simulink model "attitude_template_link"  (R2019a)
settings: Solver=ode1  StartTime=0.0  StopTime=inf  FixedStep=1/1000  RelTol=1e-3
PreLoadFcn:
  | x_setpoint_NED = 0;
  | y_setpoint_NED = 0;
  | z_setpoint_NED = 0;
  | vx_setpoint_NED = 0;
  | vy_setpoint_NED = 0;
  | vz_setpoint_NED = 0;
  | afx_setpoint_NED = 0;
  | afy_setpoint_NED = 0;
  | afz_setpoint_NED = 0;
  | yaw_setpoint_NED = 0;
  | yawrate_setpoint_NED = 0;
  | selected_mission = 1;
  | pitch_ol = 0;
  | roll_ol = 0;
  | yaw_ol = 0;
  | theta_xz_setpoint = 0;
  | thrustVal = 0;
  | parentThruster = 0;
  | 
  | return_com = 0;
  | takeoff_com = 0;
  | mission_com = 0;
  | hold_com = 0;
  | land_com = 0;
  | direct_com = 0;
  | origin_update = 0;
InitFcn:
  | x_setpoint_NED = 0;
  | y_setpoint_NED = 0;
  | z_setpoint_NED = 0;
  | vx_setpoint_NED = 0;
  | vy_setpoint_NED = 0;
  | vz_setpoint_NED = 0;
  | afx_setpoint_NED = 0;
  | afy_setpoint_NED = 0;
  | afz_setpoint_NED = 0;
  | yaw_setpoint_NED = 0;
  | yawrate_setpoint_NED = 0;
  | selected_mission = 1;
  | pitch_ol = 0;
  | roll_ol = 0;
  | yaw_ol = 0;
  | theta_xz_setpoint = 0;
  | thrustVal = 0;
  | parentThruster = 0;
  | 
  | return_com = 0;
  | takeoff_com = 0;
  | mission_com = 0;
  | hold_com = 0;
  | land_com = 0;
  | direct_com = 0;
  | origin_update = 0;
StartFcn:
  | yaw_ol = 0;
undefined symbols (not defined in the file or in its folder): f, Object1, Object2, origin_pos_yaw, pitch, roll, roll_input, Standard_Devices, time_usec, UDP_Protocol, x, y, yaw, z
libraries: simulink_extras x17, simulink x3, sldrtlib x3, instrumentlib x1
settings Model: Creator=Admin  LastModifiedBy=viconadmin
settings DataIOCC: SaveFormat=StructureWithTime  ReturnWorkspaceOutputs=off
settings DebuggingCC: ArithmeticOperatorsInVariantConditions=warning
settings SFSimCC: SimUseLocalCustomCode=off
settings RTWCC: RTWUseLocalCustomCode=off
settings CodeAppCC: StateflowObjectComments=on

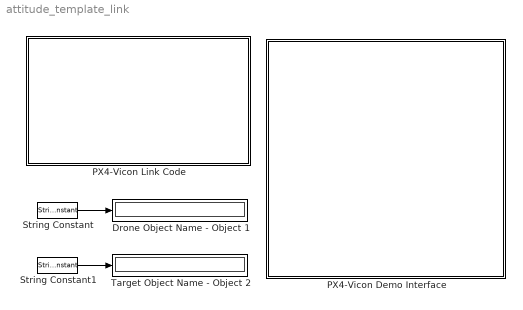
== system attitude_template_link ==
  Drone Object Name - Object 1 : Display
  PX4-Vicon Demo Interface : Subsystem
  PX4-Vicon Link Code : Subsystem
  String Constant : StringConstant  String=Object1
  String Constant1 : StringConstant  String=Object2
  Target Object Name - Object 2 : Display
  wires:
  String Constant/1 -> Drone Object Name - Object 1/1
  String Constant1/1 -> Target Object Name - Object 2/1

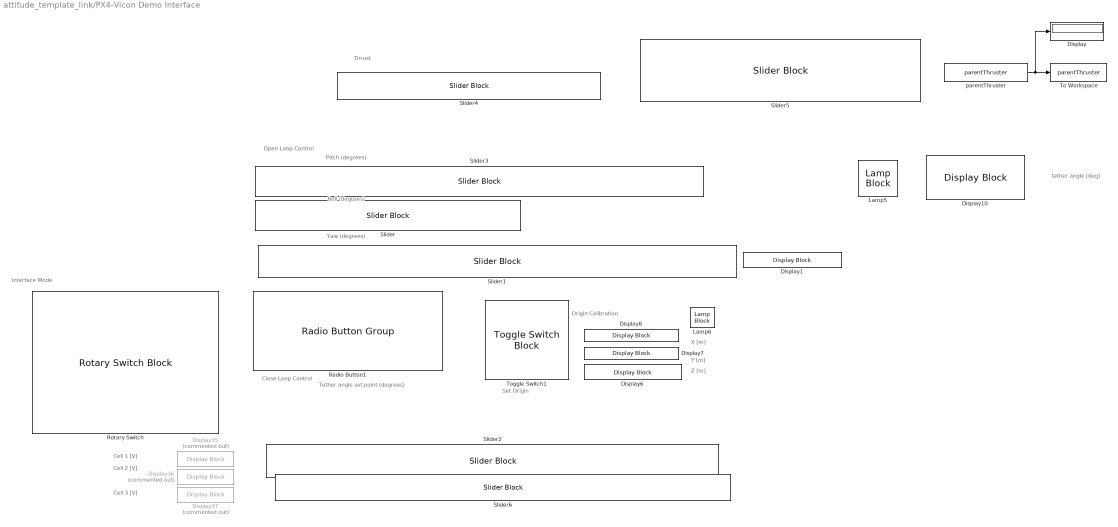
== system attitude_template_link/PX4-Vicon Demo Interface ==
  note: Thrust
  note: Roll (degrees)
  note: Yaw (degrees)
  note: Pitch (degrees)
  note: Interface Mode
  note: Close Loop Control
  note: Cell 1 [V]
  note: Cell 3 [V]
  note: Cell 2 [V]
  note: Set Origin
  note: X [m]
  note: Y [m]
  note: Z [m]
  note: Origin Calibration
  note: Open Loop Control
  note: Tether angle set point (degrees)
  note: tether angle [deg]
  Display : Display
  Display{1,6..8,10} (5 alike) : DisplayBlock  LabelPosition=Hide  Format=short
  Display35 : DisplayBlock  Commented=on  LabelPosition=Hide  Format=short
  Display36 : DisplayBlock  Commented=on  LabelPosition=Hide  Format=short
  Display37 : DisplayBlock  Commented=on  LabelPosition=Hide  Format=short
  Lamp5 : LampBlock
  Lamp6 : LampBlock  LabelPosition=Hide
  Radio Button1 : RadioButtonGroup  LabelPosition=Hide  SelectedLabel=DONT  ButtonGroupName=Select Desired Control
      settings: Values={{'DONT', 'CL control', 'OL Control'}, [1 2 3]}
  Rotary Switch : RotarySwitchBlock  LabelPosition=Hide
      settings: Values={{'Hold Origin', 'Follow', 'Other'}, [1 2 3]}
  Slider : SliderBlock  LabelPosition=Hide  ScaleMin=-25  ScaleMax=25
  Slider1 : SliderBlock  LabelPosition=Hide  ScaleMin=-180  ScaleMax=180  TickInterval=10
  Slider2 : SliderBlock  LabelPosition=Hide  ScaleMin=-30  ScaleMax=60
  Slider3 : SliderBlock  LabelPosition=Hide  ScaleMin=-25  ScaleMax=60  TickInterval=5
  Slider4 : SliderBlock  LabelPosition=Hide  ScaleMax=0.5  TickInterval=0.050000000000000003
  Slider5 : SliderBlock  ScaleMax=60  TickInterval=5
  Slider6 : SliderBlock  LabelPosition=Hide  ScaleMin=-30  ScaleMax=30
  To Workspace : ToWorkspace  VariableName=parentThruster  SaveFormat=Timeseries  SampleTime=-1
  Toggle Switch1 : ToggleSwitchBlock  LabelPosition=Hide
      settings: Values={{'No action', 'Set Origin'}, [0 1]}
  parentThruster : Constant  Value=parentThruster
  wires:
  parentThruster/1 -> Display/1, To Workspace/1

== system attitude_template_link/PX4-Vicon Link Code ==
  note: MAVLink PX4 Interface Telemetry
  note: MAVLink PX4 Interface Motion Capture
  Data Manipulation : Subsystem
  Decode PX4  Telemetry Data - MAVLink : S-Function  FunctionName=sfun_decode_mavlink  SFunctionDeploymentMode=off  EnableBusSupport=off
  Mavlink Encoded - UDP Packet Output : sldrtlib/Packet Output  SampleTime=1/50  MaxMissedTicks=inf  ShowMissedTicks=off  YieldWhenWaiting=off  DrvName=Standard_Devices/UDP_Protocol  DrvAddress=14551  DrvOptions=[0 14556 48 46 48 46 48 46 48 0 0 0 0 0 0 0 0 0 0 0 0 0 0 0 0 0 0 0 0 0 0 0 0 0 0 0 0 0 0 0 0 0 0 0 0 0 0 0 0 0 0 0 0 0 0 0 0 0 0 0 0 0 0 0 0 0 0 0 0 0 0 0 0 0 0 0 0 0 0 0 0 0 0 0 0 0 0 0 0 0 0 0 0 0 0 0 0 0 0 0 0 0 0 0 0 0 0 0 0 0 0 0 0 0 0 0 0 0 0 0 0 0 0 0 0 0 0 0 0 0 0 0 0 0 0 0 0 0 0 0 0 0 0 0 0 0 0 0 0 0 0 0 0 0 0 0 0 0 0 0 0 0 0 0 0 0 0 0 0 0 0 0 0 0 0 0 0 0 0 0 0 0 0 0 0 0 0 0 0 0 0 0 0 0 0 0 0 0 0 0 0 0 0 0 0 0 0 0 0 0 0 0 0 0 0 0 0 0 0 0 0 0 0 0 0 0 0 0 0 0 0 0 0 0 0 0 0 0 0 0 0 0 0 0 0 0 0 0 0 0 0 0 0 0 0 0]  PacketSize=51  DataTypes='51*uint8'  ShowReady=off  ShowError=off  PacketID=1  ByteOrder=1  InitialValue=[]  FinalValue=[]
      settings: AttributesFormatString=UDP Protocol [14551]  SourceProductName=Simulink Desktop Real-Time
  Mavlink Encoded - UDP Packet Output1 : sldrtlib/Packet Output  SampleTime=1/50  MaxMissedTicks=inf  ShowMissedTicks=off  YieldWhenWaiting=off  DrvName=Standard_Devices/UDP_Protocol  DrvAddress=14551  DrvOptions=[0 14556 48 46 48 46 48 46 48 0 0 0 0 0 0 0 0 0 0 0 0 0 0 0 0 0 0 0 0 0 0 0 0 0 0 0 0 0 0 0 0 0 0 0 0 0 0 0 0 0 0 0 0 0 0 0 0 0 0 0 0 0 0 0 0 0 0 0 0 0 0 0 0 0 0 0 0 0 0 0 0 0 0 0 0 0 0 0 0 0 0 0 0 0 0 0 0 0 0 0 0 0 0 0 0 0 0 0 0 0 0 0 0 0 0 0 0 0 0 0 0 0 0 0 0 0 0 0 0 0 0 0 0 0 0 0 0 0 0 0 0 0 0 0 0 0 0 0 0 0 0 0 0 0 0 0 0 0 0 0 0 0 0 0 0 0 0 0 0 0 0 0 0 0 0 0 0 0 0 0 0 0 0 0 0 0 0 0 0 0 0 0 0 0 0 0 0 0 0 0 0 0 0 0 0 0 0 0 0 0 0 0 0 0 0 0 0 0 0 0 0 0 0 0 0 0 0 0 0 0 0 0 0 0 0 0 0 0 0 0 0 0 0 0 0 0 0 0 0 0 0 0 0 0 0 0]  PacketSize=44  DataTypes='44*uint8'  ShowReady=off  ShowError=off  PacketID=1  ByteOrder=1  InitialValue=[]  FinalValue=[]
      settings: AttributesFormatString=UDP Protocol [14551]  SourceProductName=Simulink Desktop Real-Time
  Packet Input : sldrtlib/Packet Input  SampleTime=1/50  MaxMissedTicks=inf  ShowMissedTicks=off  YieldWhenWaiting=off  DrvName=Standard_Devices/UDP_Protocol  DrvAddress=14551  DrvOptions=[0 14556 48 46 48 46 48 46 48 0 0 0 0 0 0 0 0 0 0 0 0 0 0 0 0 0 0 0 0 0 0 0 0 0 0 0 0 0 0 0 0 0 0 0 0 0 0 0 0 0 0 0 0 0 0 0 0 0 0 0 0 0 0 0 0 0 0 0 0 0 0 0 0 0 0 0 0 0 0 0 0 0 0 0 0 0 0 0 0 0 0 0 0 0 0 0 0 0 0 0 0 0 0 0 0 0 0 0 0 0 0 0 0 0 0 0 0 0 0 0 0 0 0 0 0 0 0 0 0 0 0 0 0 0 0 0 0 0 0 0 0 0 0 0 0 0 0 0 0 0 0 0 0 0 0 0 0 0 0 0 0 0 0 0 0 0 0 0 0 0 0 0 0 0 0 0 0 0 0 0 0 0 0 0 0 0 0 0 0 0 0 0 0 0 0 0 0 0 0 0 0 0 0 0 0 0 0 0 0 0 0 0 0 0 0 0 0 0 0 0 0 0 0 0 0 0 0 0 0 0 0 0 0 0 0 0 0 0 0 0 0 0 0 0 0 0 0 0 0 0 0 0 0 0 0 0]  PacketSize=280  DataTypes='280*uint8'  ShowReady=off  ShowError=off  PacketID=1  ByteOrder=1  ShowTimestamp=off
      settings: AttributesFormatString=UDP Protocol [14551]  SourceProductName=Simulink Desktop Real-Time
  Rate Transition : RateTransition
  Rate Transition1 : RateTransition
  Vicon Stream - UDP Packet Receive : instrumentlib/UDP Receive  Priority=3  Host=localhost  Port=9090  LocalPort=51001  EnablePortSharing=off  GetLatestData=off  DataSize=256  DataType=uint8  ASCIIFormatting=%f,  Terminator=LF  ByteOrder=BigEndian  EnableBlockingMode=off  Timeout=inf  SampleTime=-1  LocalAddress=0.0.0.0
      settings: SourceProductName=Instrument Control Toolbox
  Visualize Telemetry Data : Subsystem
  wires:
  Data Manipulation/1(Encoded_Setpoints_Output) -> Rate Transition/1
  Rate Transition/1 -> Mavlink Encoded - UDP Packet Output/1
  Packet Input/1 -> Decode PX4  Telemetry Data - MAVLink/1
  Vicon Stream - UDP Packet Receive/1 -> Data Manipulation/1(vicon_data_input)
  Vicon Stream - UDP Packet Receive/2 -> Data Manipulation/2(status)
  Decode PX4  Telemetry Data - MAVLink/2 -> Visualize Telemetry Data/2(msg_battery_status)
  Rate Transition1/1 -> Mavlink Encoded - UDP Packet Output1/1
  Data Manipulation/2(Encoded_Mocap_Output) -> Rate Transition1/1
  Decode PX4  Telemetry Data - MAVLink/1 -> Visualize Telemetry Data/1(msg_attitude)

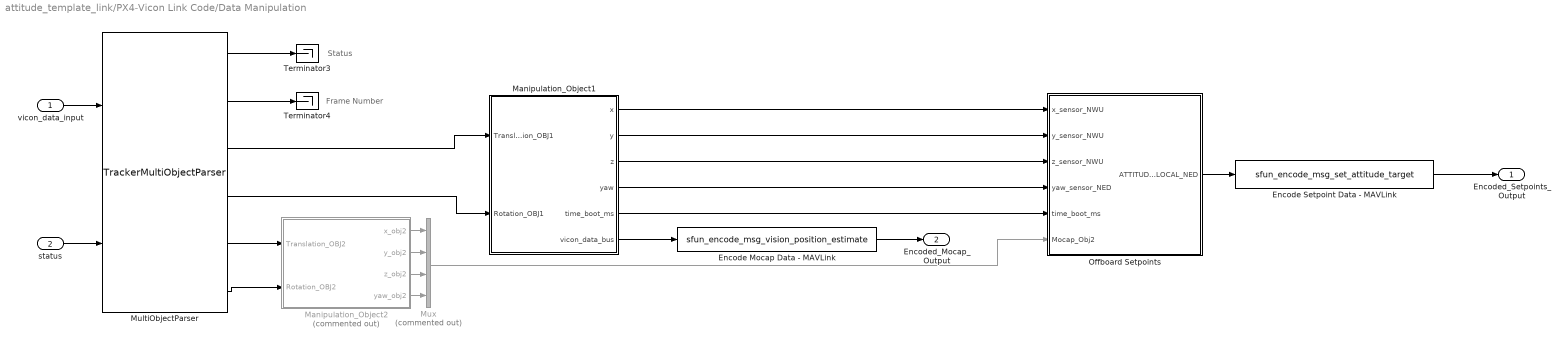
== system attitude_template_link/PX4-Vicon Link Code/Data Manipulation ==
  note: Status
  note: Frame Number
  vicon_data_input : Inport
  status : Inport  Port=2
  "Encode Mocap Data - MAVLink " : S-Function  FunctionName=sfun_encode_msg_vision_position_estimate  SFunctionDeploymentMode=off  EnableBusSupport=off
  Encode Setpoint Data - MAVLink : S-Function  FunctionName=sfun_encode_msg_set_attitude_target  SFunctionDeploymentMode=off  EnableBusSupport=off
  Manipulation_Object1 : Subsystem
  Manipulation_Object2 : Subsystem  Commented=on
  MultiObjectParser : S-Function  Tag=Data_Parser_Multi  FunctionName=TrackerMultiObjectParser  Parameters=Object1,Object2  SFunctionModules=TrackerMultiObjectParser  SFunctionDeploymentMode=off  EnableBusSupport=off
      settings: AttributesFormatString=Data_Parser_Multi
  Mux : Mux  Commented=on
  Offboard Setpoints : Subsystem
  Terminator3 : Terminator
  Terminator4 : Terminator
  Encoded_Setpoints_Output : Outport
  Encoded_Mocap_Output : Outport  Port=2
  wires:
  MultiObjectParser/3 -> Manipulation_Object1/1(Translation_OBJ1)
  MultiObjectParser/2 -> Terminator4/1
  Manipulation_Object1/1(x) -> Offboard Setpoints/1(x_sensor_NWU)
  MultiObjectParser/1 -> Terminator3/1
  Manipulation_Object1/6(vicon_data_bus) -> "Encode Mocap Data - MAVLink "/1
  MultiObjectParser/5 -> Manipulation_Object2/1(Translation_OBJ2)
  MultiObjectParser/6 -> Manipulation_Object2/2(Rotation_OBJ2)
  MultiObjectParser/4 -> Manipulation_Object1/2(Rotation_OBJ1)
  Manipulation_Object1/4(yaw) -> Offboard Setpoints/4(yaw_sensor_NED)
  status/1 -> MultiObjectParser/2
  Manipulation_Object1/3(z) -> Offboard Setpoints/3(z_sensor_NWU)
  Manipulation_Object1/2(y) -> Offboard Setpoints/2(y_sensor_NWU)
  "Encode Mocap Data - MAVLink "/1 -> Encoded_Mocap_Output/1
  vicon_data_input/1 -> MultiObjectParser/1
  Manipulation_Object1/5(time_boot_ms) -> Offboard Setpoints/5(time_boot_ms)
  Offboard Setpoints/1(ATTITUDE_TARGET_LOCAL_NED) -> Encode Setpoint Data - MAVLink/1
  Encode Setpoint Data - MAVLink/1 -> Encoded_Setpoints_Output/1
  Manipulation_Object2/4(yaw_obj2) -> Mux/4
  Manipulation_Object2/3(z_obj2) -> Mux/3
  Manipulation_Object2/2(y_obj2) -> Mux/2
  Manipulation_Object2/1(x_obj2) -> Mux/1
  Mux/1 -> Offboard Setpoints/6(Mocap_Obj2)

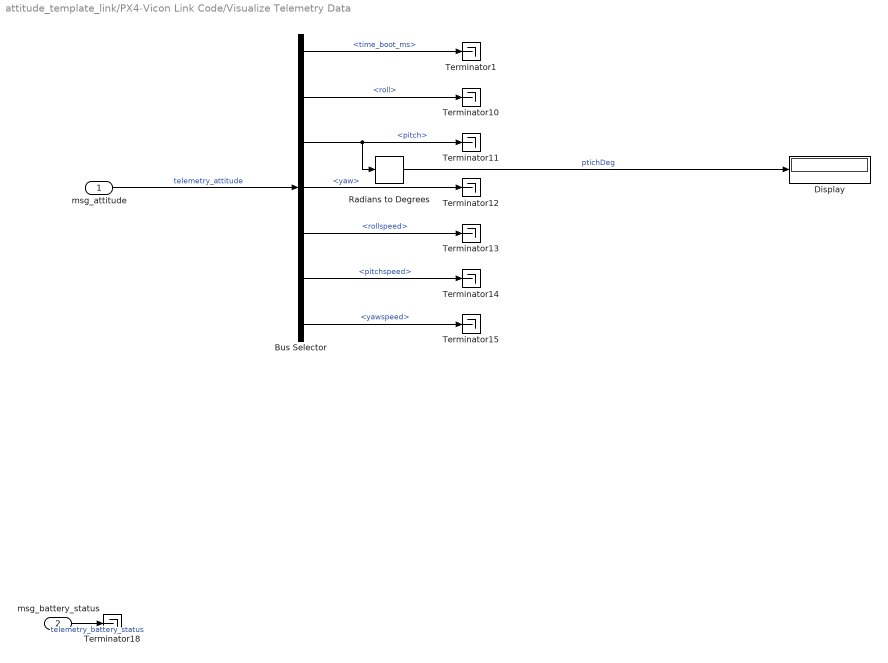
== system attitude_template_link/PX4-Vicon Link Code/Visualize Telemetry Data ==
  msg_attitude : Inport
  msg_battery_status : Inport  Port=2
  Bus Selector : BusSelector  OutputSignals=time_boot_ms,roll,pitch,yaw,rollspeed,pitchspeed,yawspeed
  Display : Display
  Radians to Degrees : simulink_extras/Transformations/Radians to Degrees
  Terminator{1,10..15,18} (8 alike) : Terminator
  wires:
  Bus Selector/7 -> Terminator15/1  "<yawspeed>"
  Bus Selector/5 -> Terminator13/1  "<rollspeed>"
  Bus Selector/2 -> Terminator10/1  "<roll>"
  Bus Selector/1 -> Terminator1/1  "<time_boot_ms>"
  Bus Selector/4 -> Terminator12/1  "<yaw>"
  Bus Selector/3 -> Radians to Degrees/1, Terminator11/1  "<pitch>"
  Bus Selector/6 -> Terminator14/1  "<pitchspeed>"
  msg_attitude/1 -> Bus Selector/1  "telemetry_attitude"
  msg_battery_status/1 -> Terminator18/1  "telemetry_battery_status"
  Radians to Degrees/1 -> Display/1  "ptichDeg"

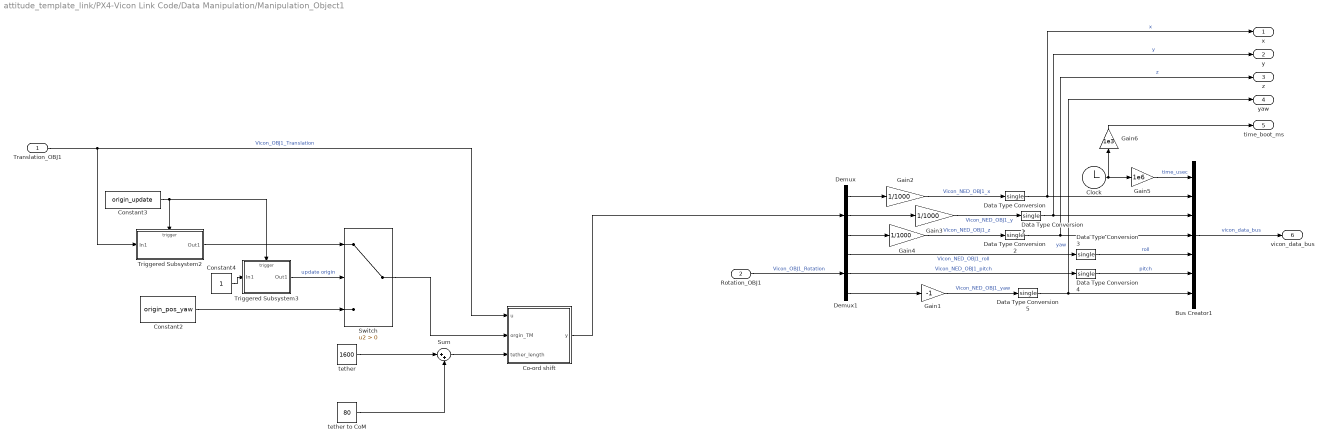
== system attitude_template_link/PX4-Vicon Link Code/Data Manipulation/Manipulation_Object1 ==
  Translation_OBJ1 : Inport
  Rotation_OBJ1 : Inport  Port=2
  Bus Creator1 : BusCreator  Inputs=time_usec,x,y,z,roll,pitch,yaw  OutDataTypeStr=Bus: mavlink_vision_position_estimate_t
  Clock : Clock
      settings: Decimation=100
  Co-ord shift : MATLAB Function  TreatAsAtomicUnit=on
  Constant2 : Constant  Value=origin_pos_yaw
  Constant3 : Constant  Value=origin_update
  Constant4 : Constant
  Data Type Conversion{,1..5} (6 alike) : DataTypeConversion  OutDataTypeStr=single
  Demux : Demux  Outputs=3
  Demux1 : Demux  Outputs=3
  Gain1 : Gain  Gain=-1  OutDataTypeStr=Inherit: Same as input
  Gain2 : Gain  Gain=1/1000  OutDataTypeStr=double
  Gain3 : Gain  Gain=1/1000  OutDataTypeStr=double
  Gain4 : Gain  Gain=1/1000  OutDataTypeStr=double
  Gain5 : Gain  Gain=1e6  OutDataTypeStr=double
  Gain6 : Gain  Gain=1e3  OutDataTypeStr=double
  Sum : Sum  Inputs=|++
  Switch : Switch  Criteria=u2 > Threshold
  Triggered Subsystem2 : Subsystem  TreatAsAtomicUnit=on
  Triggered Subsystem3 : Subsystem  TreatAsAtomicUnit=on
  tether : Constant  Value=1600
  tether to CoM : Constant  Value=80
  x : Outport
  y : Outport  Port=2
  z : Outport  Port=3
  yaw : Outport  Port=4
  time_boot_ms : Outport  Port=5
  vicon_data_bus : Outport  Port=6
  wires:
  Data Type Conversion1/1 -> y/1, Bus Creator1/3  "y"
  Bus Creator1/1 -> vicon_data_bus/1  "vicon_data_bus"
  Data Type Conversion5/1 -> yaw/1, Bus Creator1/7  "yaw"
  Gain4/1 -> Data Type Conversion2/1  "Vicon_NED_OBJ1_z"
  Gain1/1 -> Data Type Conversion5/1  "Vicon_NED_OBJ1_yaw"
  Data Type Conversion4/1 -> Bus Creator1/6  "pitch"
  Gain2/1 -> Data Type Conversion/1  "Vicon_NED_OBJ1_x"
  Gain3/1 -> Data Type Conversion1/1  "Vicon_NED_OBJ1_y"
  Demux/3 -> Gain4/1
  Data Type Conversion2/1 -> z/1, Bus Creator1/4  "z"
  Gain5/1 -> Bus Creator1/1  "time_usec"
  Demux1/2 -> Data Type Conversion4/1  "Vicon_NED_OBJ1_pitch"
  Data Type Conversion/1 -> x/1, Bus Creator1/2  "x"
  Data Type Conversion3/1 -> Bus Creator1/5  "roll"
  Demux1/1 -> Data Type Conversion3/1  "Vicon_NED_OBJ1_roll"
  Clock/1 -> Gain6/1, Gain5/1
  Demux1/3 -> Gain1/1
  Gain6/1 -> time_boot_ms/1
  Demux/2 -> Gain3/1
  Demux/1 -> Gain2/1
  Translation_OBJ1/1 -> Co-ord shift/1(u), Triggered Subsystem2/1(In1)  "Vicon_OBJ1_Translation"
  Rotation_OBJ1/1 -> Demux1/1  "Vicon_OBJ1_Rotation"
  Constant3/1 -> Triggered Subsystem3/Trigger, Triggered Subsystem2/Trigger
  Constant4/1 -> Triggered Subsystem3/1(In1)
  Triggered Subsystem3/1(Out1) -> Switch/2  "update origin"
  Constant2/1 -> Switch/3
  Triggered Subsystem2/1(Out1) -> Switch/1
  tether/1 -> Sum/1
  Co-ord shift/1(y) -> Demux/1
  Switch/1 -> Co-ord shift/2(orgin_TM)
  tether to CoM/1 -> Sum/2
  Sum/1 -> Co-ord shift/3(tether_length)

== system attitude_template_link/PX4-Vicon Link Code/Data Manipulation/Manipulation_Object2 ==
  Translation_OBJ2 : Inport
  Rotation_OBJ2 : Inport  Port=2
  Demux : Demux  Outputs=3
  Demux1 : Demux  Outputs=3
  Gain1 : Gain  Gain=-1  OutDataTypeStr=Inherit: Same as input
  Gain3 : Gain  Gain=-1  OutDataTypeStr=double
  Gain4 : Gain  Gain=-1  OutDataTypeStr=double
  Terminator3 : Terminator
  Terminator4 : Terminator
  x_obj2 : Outport  VectorParamsAs1DForOutWhenUnconnected=on
  y_obj2 : Outport  Port=2  VectorParamsAs1DForOutWhenUnconnected=on
  z_obj2 : Outport  Port=3  VectorParamsAs1DForOutWhenUnconnected=on
  yaw_obj2 : Outport  Port=4  VectorParamsAs1DForOutWhenUnconnected=on
  wires:
  Gain1/1 -> yaw_obj2/1  "Vicon_NED_OBJ2_yaw"
  Demux1/2 -> Terminator4/1  "Vicon_NED_OBJ2_pitch"
  Demux/3 -> Gain4/1
  Demux1/1 -> Terminator3/1  "Vicon_NED_OBJ2_roll"
  Demux1/3 -> Gain1/1
  Demux/2 -> Gain3/1
  Translation_OBJ2/1 -> Demux/1  "Vicon_OBJ2_Translation"
  Rotation_OBJ2/1 -> Demux1/1  "Vicon_OBJ2_Rotation"
  Demux/1 -> x_obj2/1  "Vicon_NED_OBJ2_x"
  Gain3/1 -> y_obj2/1  "Vicon_NED_OBJ2_y"
  Gain4/1 -> z_obj2/1  "Vicon_NE_OBJ2_z"

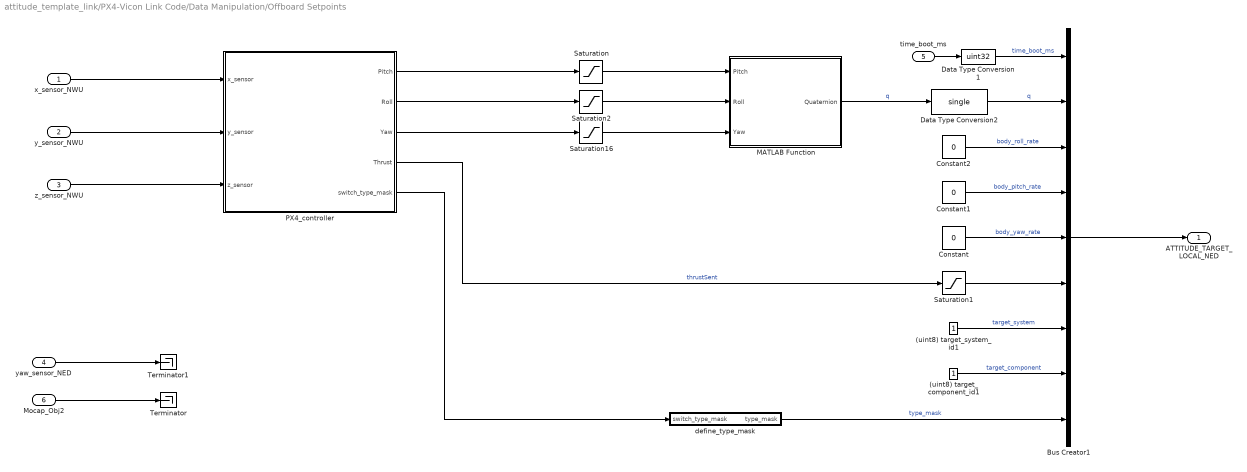
== system attitude_template_link/PX4-Vicon Link Code/Data Manipulation/Offboard Setpoints ==
  x_sensor_NWU : Inport
  y_sensor_NWU : Inport  Port=2
  z_sensor_NWU : Inport  Port=3
  yaw_sensor_NED : Inport  Port=4
  time_boot_ms : Inport  Port=5
  Mocap_Obj2 : Inport  Port=6
  (uint8) target_component_id1 : Constant  OutDataTypeStr=uint8
  (uint8) target_system_id1 : Constant  OutDataTypeStr=uint8
  Bus Creator1 : BusCreator  Inputs=9  OutDataTypeStr=Bus: mavlink_set_attitude_target_t
  Constant : Constant  Value=0  OutDataTypeStr=single
  Constant1 : Constant  Value=0  OutDataTypeStr=single
  Constant2 : Constant  Value=0  OutDataTypeStr=single
  Data Type Conversion1 : DataTypeConversion  OutDataTypeStr=uint32
  Data Type Conversion2 : DataTypeConversion  OutDataTypeStr=single
  MATLAB Function : MATLAB Function  TreatAsAtomicUnit=on
  PX4_controller : Subsystem
  Saturation : Saturate  UpperLimit=deg2rad(60)  LowerLimit=deg2rad(-60)
  Saturation1 : Saturate  UpperLimit=0.55  LowerLimit=0
  Saturation16 : Saturate  UpperLimit=deg2rad(180)  LowerLimit=deg2rad(-180)
  Saturation2 : Saturate  UpperLimit=deg2rad(40)  LowerLimit=deg2rad(-40)
  Terminator : Terminator
  Terminator1 : Terminator
  define_type_mask : Subsystem
  ATTITUDE_TARGET_LOCAL_NED : Outport
  wires:
  (uint8) target_system_id1/1 -> Bus Creator1/7  "target_system"
  time_boot_ms/1 -> Data Type Conversion1/1
  Bus Creator1/1 -> ATTITUDE_TARGET_LOCAL_NED/1
  Data Type Conversion2/1 -> Bus Creator1/2  "q"
  PX4_controller/4(Thrust) -> Saturation1/1  "thrustSent"
  Constant/1 -> Bus Creator1/5  "body_yaw_rate"
  Constant2/1 -> Bus Creator1/3  "body_roll_rate"
  Constant1/1 -> Bus Creator1/4  "body_pitch_rate"
  (uint8) target_component_id1/1 -> Bus Creator1/8  "target_component"
  Data Type Conversion1/1 -> Bus Creator1/1  "time_boot_ms"
  define_type_mask/1(type_mask) -> Bus Creator1/9  "type_mask"
  PX4_controller/5(switch_type_mask) -> define_type_mask/1(switch_type_mask)
  x_sensor_NWU/1 -> PX4_controller/1(x_sensor)
  y_sensor_NWU/1 -> PX4_controller/2(y_sensor)
  z_sensor_NWU/1 -> PX4_controller/3(z_sensor)
  PX4_controller/1(Pitch) -> Saturation/1
  PX4_controller/2(Roll) -> Saturation2/1
  Mocap_Obj2/1 -> Terminator/1
  PX4_controller/3(Yaw) -> Saturation16/1
  Saturation2/1 -> MATLAB Function/2(Roll)
  Saturation1/1 -> Bus Creator1/6
  Saturation16/1 -> MATLAB Function/3(Yaw)
  Saturation/1 -> MATLAB Function/1(Pitch)
  MATLAB Function/1(Quaternion) -> Data Type Conversion2/1  "q"
  yaw_sensor_NED/1 -> Terminator1/1

== system attitude_template_link/PX4-Vicon Link Code/Data Manipulation/Manipulation_Object1/Triggered Subsystem2 ==
  In1 : Inport
  Trigger : TriggerPort  VariantControl=Variant  InitialTriggerSignalState=zero
  Out1 : Outport  VectorParamsAs1DForOutWhenUnconnected=on
  wires:
  In1/1 -> Out1/1

== system attitude_template_link/PX4-Vicon Link Code/Data Manipulation/Manipulation_Object1/Triggered Subsystem3 ==
  In1 : Inport
  Trigger : TriggerPort  VariantControl=Variant  InitialTriggerSignalState=zero
  Out1 : Outport  VectorParamsAs1DForOutWhenUnconnected=on
  wires:
  In1/1 -> Out1/1

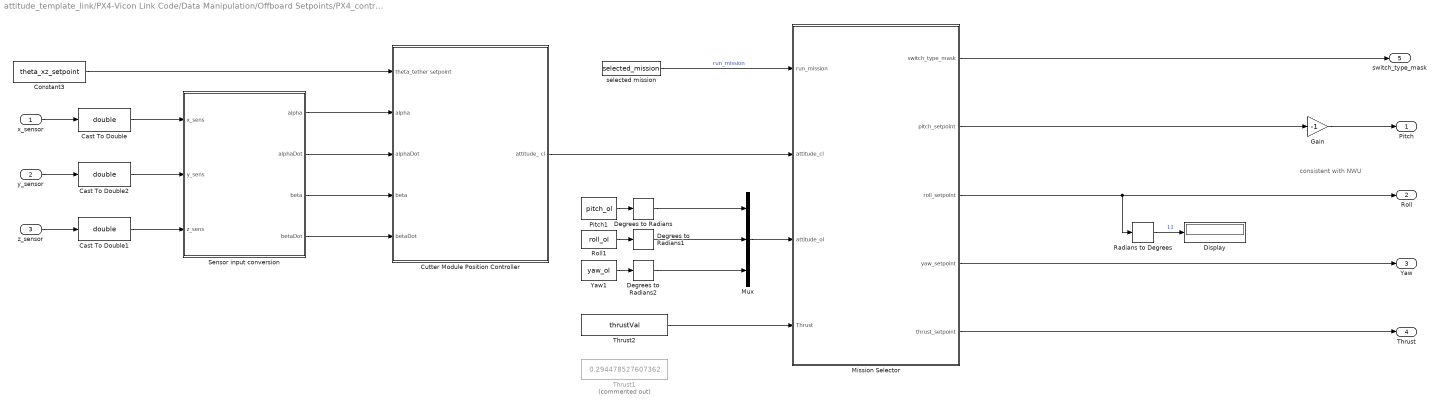
== system attitude_template_link/PX4-Vicon Link Code/Data Manipulation/Offboard Setpoints/PX4_controller ==
  note: consistent with NWU
  x_sensor : Inport
  y_sensor : Inport  Port=2
  z_sensor : Inport  Port=3
  Cast To Double : DataTypeConversion  OutDataTypeStr=double
  Cast To Double1 : DataTypeConversion  OutDataTypeStr=double
  Cast To Double2 : DataTypeConversion  OutDataTypeStr=double
  Constant3 : Constant  Value=theta_xz_setpoint
  Cutter Module Position Controller : Subsystem
  Degrees to Radians : simulink_extras/Transformations/Degrees to Radians
  Degrees to Radians1 : simulink_extras/Transformations/Degrees to Radians
  Degrees to Radians2 : simulink_extras/Transformations/Degrees to Radians
  Display : Display
  Gain : Gain  Gain=-1
  Mission Selector : Subsystem
  Mux : Mux  Inputs=3
  Pitch1 : Constant  Value=pitch_ol  OutDataTypeStr=single  SampleTime=-1
  Radians to Degrees : simulink_extras/Transformations/Radians to Degrees
  Roll1 : Constant  Value=roll_ol  OutDataTypeStr=single  SampleTime=-1
  Sensor input conversion : Subsystem
  Thrust1 : Constant  Commented=on  Value=0.294478527607362  OutDataTypeStr=double
  Thrust2 : Constant  Value=thrustVal  OutDataTypeStr=single  SampleTime=-1
  Yaw1 : Constant  Value=yaw_ol  OutDataTypeStr=single  SampleTime=-1
  selected mission : Constant  Value=selected_mission  OutDataTypeStr=single
  Pitch : Outport  PortDimensions=1
  Roll : Outport  Port=2  PortDimensions=1
  Yaw : Outport  Port=3  PortDimensions=1
  Thrust : Outport  Port=4  PortDimensions=1
  switch_type_mask : Outport  Port=5
  wires:
  y_sensor/1 -> Cast To Double2/1
  x_sensor/1 -> Cast To Double/1
  z_sensor/1 -> Cast To Double1/1
  Constant3/1 -> Cutter Module Position Controller/1(theta_tether setpoint)
  selected mission/1 -> Mission Selector/1(run_mission)  "run_mission"
  Mission Selector/1(switch_type_mask) -> switch_type_mask/1
  Thrust2/1 -> Mission Selector/4(Thrust)
  Yaw1/1 -> Degrees to Radians2/1
  Roll1/1 -> Degrees to Radians1/1
  Degrees to Radians2/1 -> Mux/3
  Degrees to Radians1/1 -> Mux/2
  Pitch1/1 -> Degrees to Radians/1
  Degrees to Radians/1 -> Mux/1
  Mission Selector/2(pitch_setpoint) -> Gain/1
  Mission Selector/5(thrust_setpoint) -> Thrust/1
  Mission Selector/4(yaw_setpoint) -> Yaw/1
  Mission Selector/3(roll_setpoint) -> Radians to Degrees/1, Roll/1
  Cutter Module Position Controller/1(attitude_ cl) -> Mission Selector/2(attitude_cl)
  Mux/1 -> Mission Selector/3(attitude_ol)
  Gain/1 -> Pitch/1
  Cast To Double/1 -> Sensor input conversion/1(x_sens)
  Sensor input conversion/1(alpha) -> Cutter Module Position Controller/2(alpha)
  Sensor input conversion/3(beta) -> Cutter Module Position Controller/4(beta)
  Cast To Double2/1 -> Sensor input conversion/2(y_sens)
  Cast To Double1/1 -> Sensor input conversion/3(z_sens)
  Sensor input conversion/2(alphaDot) -> Cutter Module Position Controller/3(alphaDot)
  Sensor input conversion/4(betaDot) -> Cutter Module Position Controller/5(betaDot)
  Radians to Degrees/1 -> Display/1  "11"

== system attitude_template_link/PX4-Vicon Link Code/Data Manipulation/Offboard Setpoints/define_type_mask ==
  note: Mappings: If any of these bits are set, the corresponding input should be ignored: bit 1: body roll rate, bit 2: body pitch rate, bit 3: body yaw rate. bit 4-bit 6: reserved, bit 7: throttle, bit 8: attitude
  switch_type_mask : Inport
  Constant : Constant  Value=7  OutDataTypeStr=uint8
  Constant1 : Constant  Value=255  OutDataTypeStr=uint8
  Merge : Merge
  Switch Case : SwitchCase  CaseConditions={1,[2,3]}  ShowDefaultCase=off
  Switch Case Action Subsystem : Subsystem  TreatAsAtomicUnit=on
  Switch Case Action Subsystem1 : Subsystem  TreatAsAtomicUnit=on
  type_mask : Outport
  wires:
  switch_type_mask/1 -> Switch Case/1
  Switch Case/1 -> Switch Case Action Subsystem/Action
  Switch Case/2 -> Switch Case Action Subsystem1/Action
  Switch Case Action Subsystem/1(Out1) -> Merge/1
  Switch Case Action Subsystem1/1(Out1) -> Merge/2
  Constant/1 -> Switch Case Action Subsystem1/1(In1)
  Constant1/1 -> Switch Case Action Subsystem/1(In1)
  Merge/1 -> type_mask/1

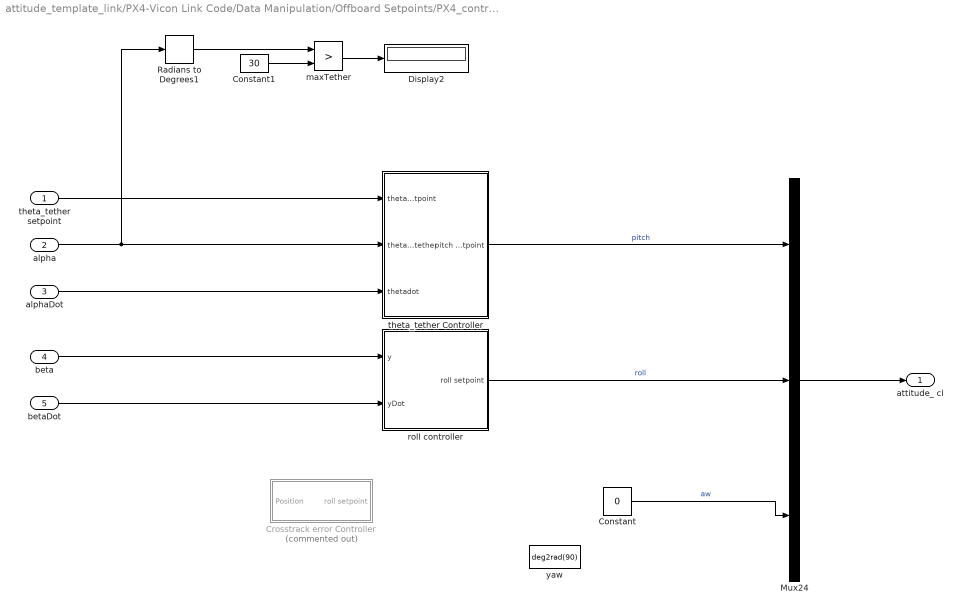
== system attitude_template_link/PX4-Vicon Link Code/Data Manipulation/Offboard Setpoints/PX4_controller/Cutter Module Position Controller ==
  theta_tether setpoint : Inport
  alpha : Inport  Port=2
  alphaDot : Inport  Port=3
  beta : Inport  Port=4
  betaDot : Inport  Port=5
  Constant : Constant  Value=0
  Constant1 : Constant  Value=30
  Crosstrack error Controller : Subsystem  Commented=on
  Display2 : Display
  Mux24 : Mux  Inputs=3
  Radians to Degrees1 : simulink_extras/Transformations/Radians to Degrees
  maxTether : RelationalOperator  Operator=>  OutDataTypeStr=boolean  RndMeth=Simplest
  roll controller : Subsystem
  theta_tether Controller : Subsystem
  yaw : Constant  Value=deg2rad(90)
  attitude_ cl : Outport
  wires:
  theta_tether setpoint/1 -> theta_tether Controller/1(theta_tether setpoint)
  Mux24/1 -> attitude_ cl/1
  alphaDot/1 -> theta_tether Controller/3(thetadot)
  betaDot/1 -> roll controller/2(yDot)
  beta/1 -> roll controller/1(y)
  maxTether/1 -> Display2/1
  Constant1/1 -> maxTether/2
  alpha/1 -> theta_tether Controller/2(theta_tether), Radians to Degrees1/1
  Radians to Degrees1/1 -> maxTether/1
  Constant/1 -> Mux24/3  "aw"
  theta_tether Controller/1(pitch setpoint) -> Mux24/1  "pitch"
  roll controller/1(roll setpoint) -> Mux24/2  "roll"

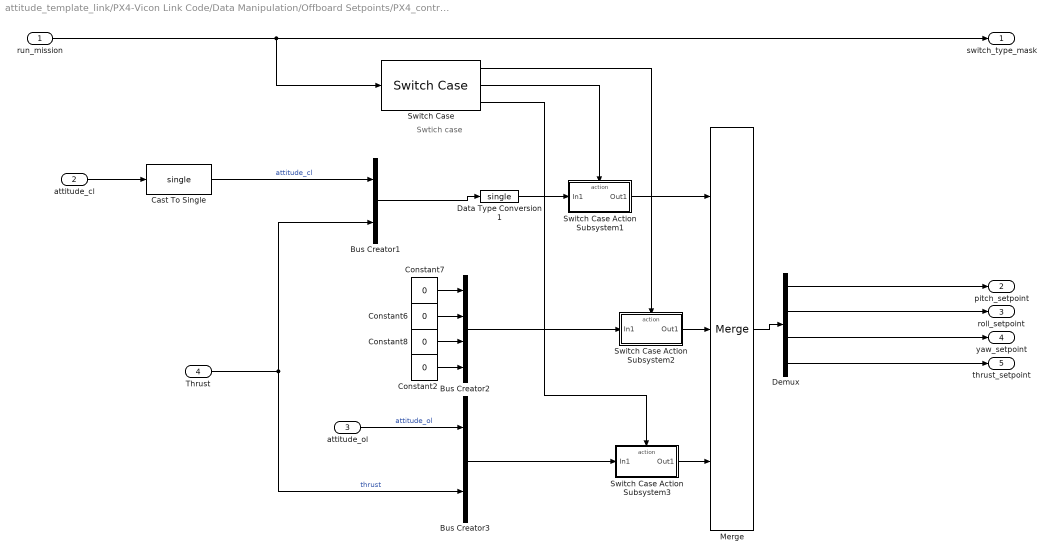
== system attitude_template_link/PX4-Vicon Link Code/Data Manipulation/Offboard Setpoints/PX4_controller/Mission Selector ==
  note: Swtich case
  run_mission : Inport
  attitude_cl : Inport  Port=2
  attitude_ol : Inport  Port=3  OutDataTypeStr=single
  Thrust : Inport  Port=4
  Bus Creator1 : BusCreator  Inputs=2
  Bus Creator2 : BusCreator  Inputs=4
  Bus Creator3 : BusCreator  Inputs=2
  Cast To Single : DataTypeConversion  OutDataTypeStr=single
  Constant{2,6..8} (4 alike) : Constant  Value=0  OutDataTypeStr=single
  Data Type Conversion1 : DataTypeConversion  OutDataTypeStr=single
  Demux : Demux
  Merge : Merge  Inputs=3
  Switch Case : SwitchCase  CaseConditions={1,2,3}  ShowDefaultCase=off
  Switch Case Action Subsystem1 : Subsystem  TreatAsAtomicUnit=on
  Switch Case Action Subsystem2 : Subsystem  TreatAsAtomicUnit=on
  Switch Case Action Subsystem3 : Subsystem  TreatAsAtomicUnit=on
  switch_type_mask : Outport
  pitch_setpoint : Outport  Port=2
  roll_setpoint : Outport  Port=3
  yaw_setpoint : Outport  Port=4
  thrust_setpoint : Outport  Port=5
  wires:
  Constant7/1 -> Bus Creator2/1
  Thrust/1 -> Bus Creator3/2, Bus Creator1/2  "thrust"
  Demux/2 -> roll_setpoint/1
  Switch Case/3 -> Switch Case Action Subsystem3/Action
  Demux/4 -> thrust_setpoint/1
  Switch Case/2 -> Switch Case Action Subsystem1/Action
  run_mission/1 -> switch_type_mask/1, Switch Case/1
  Bus Creator1/1 -> Data Type Conversion1/1
  Demux/3 -> yaw_setpoint/1
  Bus Creator3/1 -> Switch Case Action Subsystem3/1(In1)
  Bus Creator2/1 -> Switch Case Action Subsystem2/1(In1)
  attitude_ol/1 -> Bus Creator3/1  "attitude_ol"
  Data Type Conversion1/1 -> Switch Case Action Subsystem1/1(In1)
  Switch Case Action Subsystem1/1(Out1) -> Merge/1
  Merge/1 -> Demux/1
  Switch Case/1 -> Switch Case Action Subsystem2/Action
  Constant2/1 -> Bus Creator2/4
  Switch Case Action Subsystem2/1(Out1) -> Merge/2
  Switch Case Action Subsystem3/1(Out1) -> Merge/3
  Constant6/1 -> Bus Creator2/2
  Constant8/1 -> Bus Creator2/3
  attitude_cl/1 -> Cast To Single/1
  Demux/1 -> pitch_setpoint/1
  Cast To Single/1 -> Bus Creator1/1  "attitude_cl"

== system attitude_template_link/PX4-Vicon Link Code/Data Manipulation/Offboard Setpoints/PX4_controller/Sensor input conversion ==
  x_sens : Inport
  y_sens : Inport  Port=2
  z_sens : Inport  Port=3
  MATLAB Function : MATLAB Function  TreatAsAtomicUnit=on
  MATLAB Function1 : MATLAB Function  TreatAsAtomicUnit=on
  Transfer Fcn : TransferFcn  Numerator=[100 0]  Denominator=[1 100]
  Transfer Fcn1 : TransferFcn  Numerator=[100 0]  Denominator=[1 100]
  alpha : Outport
  alphaDot : Outport  Port=2
  beta : Outport  Port=3
  betaDot : Outport  Port=4
  wires:
  MATLAB Function1/1(theta_yz) -> beta/1, Transfer Fcn/1
  MATLAB Function/1(theta_xz) -> alpha/1, Transfer Fcn1/1
  z_sens/1 -> MATLAB Function1/1(z), MATLAB Function/2(z)
  x_sens/1 -> MATLAB Function/1(x)
  Transfer Fcn1/1 -> alphaDot/1
  Transfer Fcn/1 -> betaDot/1
  y_sens/1 -> MATLAB Function1/2(y)

== system attitude_template_link/PX4-Vicon Link Code/Data Manipulation/Offboard Setpoints/define_type_mask/Switch Case Action Subsystem ==
  In1 : Inport
  Action Port : ActionPort  ActionPortLabel=case [ 1 ]:
  Out1 : Outport
  wires:
  In1/1 -> Out1/1

== system attitude_template_link/PX4-Vicon Link Code/Data Manipulation/Offboard Setpoints/define_type_mask/Switch Case Action Subsystem1 ==
  In1 : Inport
  Action Port : ActionPort  ActionPortLabel=case [ 2 3 ]:
  Out1 : Outport
  wires:
  In1/1 -> Out1/1

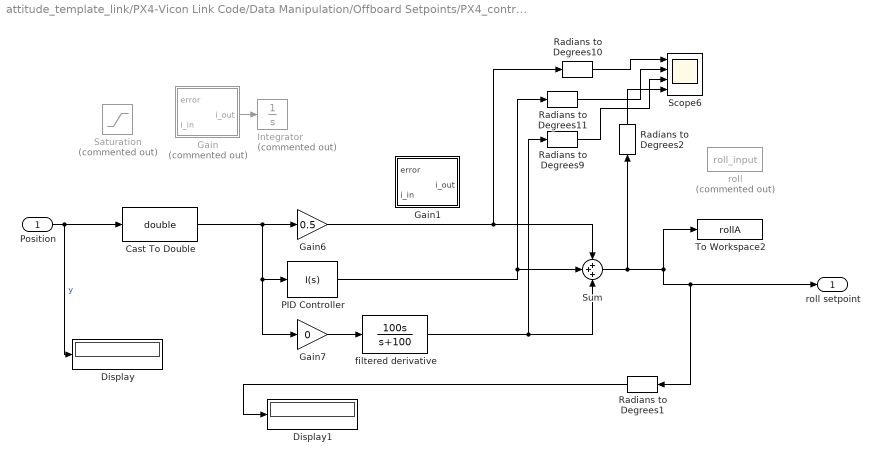
== system attitude_template_link/PX4-Vicon Link Code/Data Manipulation/Offboard Setpoints/PX4_controller/Cutter Module Position Controller/Crosstrack error Controller ==
  Position : Inport
  Cast To Double : DataTypeConversion  OutDataTypeStr=double
  Display : Display
  Display1 : Display
  Gain : MATLAB Function  Commented=on  TreatAsAtomicUnit=on
  Gain1 : MATLAB Function  TreatAsAtomicUnit=on
  Gain6 : Gain  Gain=0.5
  Gain7 : Gain  Gain=0
  Integrator : Integrator  Commented=on  UpperSaturationLimit=deg2rad(15)  LowerSaturationLimit=deg2rad(-15)
  PID Controller : simulink/Continuous/PID Controller  Controller=I  Form=Parallel  TimeDomain=Continuous-time  SampleTime=-1  IntegratorMethod=Forward Euler  FilterMethod=Forward Euler  ControllerParametersSource=internal  P=1  I=1  D=0  UseFilter=on  N=100  TunerSelectOption=Transfer Function Based (PID Tuner App)  InitialConditionSource=internal  InitialConditionForIntegrator=0  InitialConditionForFilter=0  DifferentiatorICPrevScaledInput=0  ExternalReset=none  TrackingMode=off  Kt=1  LimitOutput=on  UpperSaturationLimit=deg2rad(5)  LowerSaturationLimit=deg2rad(-5)  LinearizeAsGain=on  AntiWindupMode=clamping  Kb=1  POutMin=[]  POutMax=[]  IOutMin=[]  IOutMax=[]  DOutMin=[]  DOutMax=[]  NOutMin=[]  NOutMax=[]  SumOutMin=[]  SumOutMax=[]  SaturationOutMin=[]  SaturationOutMax=[]  PParamMin=[]  PParamMax=[]  IParamMin=[]  IParamMax=[]  DParamMin=[]  DParamMax=[]  NParamMin=[]  NParamMax=[]  KbParamMin=[]  KbParamMax=[]  KtParamMin=[]  KtParamMax=[]  KbOutMin=[]  KbOutMax=[]  KtOutMin=[]  KtOutMax=[]  IntegratorOutMin=[]  IntegratorOutMax=[]  FilterOutMin=[]  FilterOutMax=[]  SumI1OutMin=[]  SumI1OutMax=[]  SumI2OutMin=[]  SumI2OutMax=[]  SumI3OutMin=[]  SumI3OutMax=[]  SumI4OutMin=[]  SumI4OutMax=[]  SumDOutMin=[]  SumDOutMax=[]  DifferentiatorOutMin=[]  DifferentiatorOutMax=[]  FilterDiffOutCoefMin=[]  FilterDiffOutCoefMax=[]  ReciprocalOutMin=[]  ReciprocalOutMax=[]  SumDenOutMin=[]  SumDenOutMax=[]  SumNumOutMin=[]  SumNumOutMax=[]  DivideOutMin=[]  DivideOutMax=[]  IntegratorContinuousStateAttributes=''  IntegratorStateMustResolveToSignalObject=off  IntegratorRTWStateStorageClass=Auto  FilterContinuousStateAttributes=''  FilterStateMustResolveToSignalObject=off  FilterRTWStateStorageClass=Auto  ParallelPVariant=Disabled  IdealPVariant=Disabled  IVariant=InternalParameters  DVariant=Disabled  IntegratorVariant=Continuous  SatVariant=Enabled  AWVariant=ContClampingParallel  PCopyVariant=Disabled  TRVariant=Disabled  FdbkBlocksVariant=Forward  IdealPFdbkVariant=Disabled  SatFdbkVariant=Disabled  DerivativeFilterVariant=Disabled  NVariant=Disabled  NCopyVariant=Disabled_SignalSpec  FilterICVariant=Disabled  IntegratorICVariant=InternalICs  ExternalResetVariant=Disabled  TRSumVariant=Passthrough  SumFdbkVariant=Disabled  SumVariant=Passthrough_I
  Radians to Degrees{1..2,9..11} (5 alike) : simulink_extras/Transformations/Radians to Degrees
  Saturation : Saturate  Commented=on  UpperLimit=deg2rad(15)  LowerLimit=deg2rad(-15)
  Scope6 : Scope  NumInputPorts=4
  Sum : Sum  Inputs=+++
  To Workspace2 : ToWorkspace  VariableName=rollA  SampleTime=-1
      settings: Save2DSignal=2-D array (concatenate along first dimension)
  filtered derivative : TransferFcn  Numerator=[100 0]  Denominator=[1 100]
  roll : Constant  Commented=on  Value=roll_input
  roll setpoint : Outport  VectorParamsAs1DForOutWhenUnconnected=on
  wires:
  Radians to Degrees10/1 -> Scope6/1
  filtered derivative/1 -> Radians to Degrees9/1, Sum/3
  Radians to Degrees11/1 -> Scope6/2
  Position/1 -> Display/1, Cast To Double/1  "y"
  Gain6/1 -> Radians to Degrees10/1, Sum/1
  Gain7/1 -> filtered derivative/1
  Radians to Degrees9/1 -> Scope6/3
  Sum/1 -> Radians to Degrees2/1, Radians to Degrees1/1, roll setpoint/1, To Workspace2/1
  Radians to Degrees1/1 -> Display1/1
  Cast To Double/1 -> PID Controller/1, Gain7/1, Gain6/1
  Gain/1(i_out) -> Integrator/1
  Radians to Degrees2/1 -> Scope6/4
  PID Controller/1 -> Sum/2, Radians to Degrees11/1

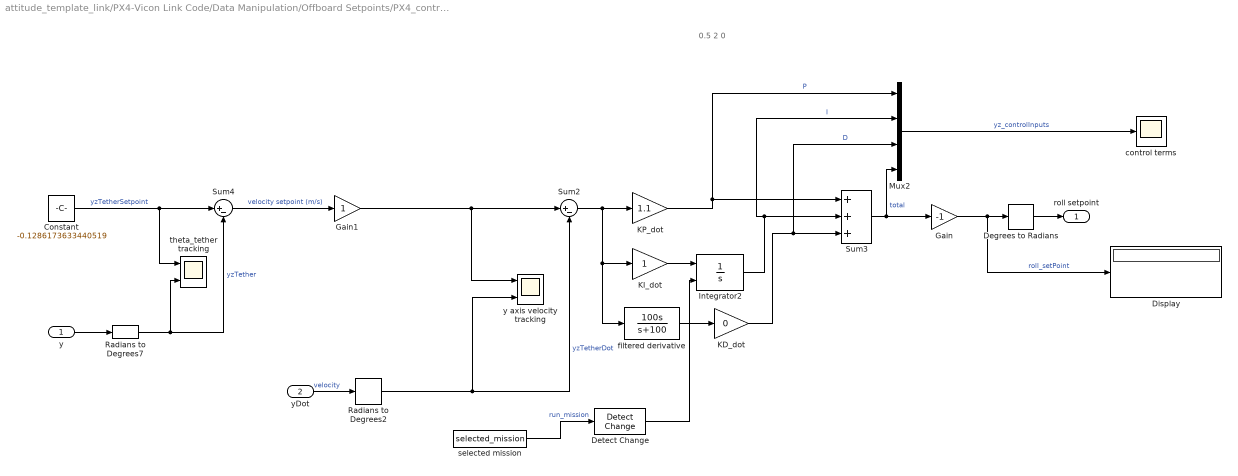
== system attitude_template_link/PX4-Vicon Link Code/Data Manipulation/Offboard Setpoints/PX4_controller/Cutter Module Position Controller/roll controller ==
  note: 0.5 2 0
  y : Inport
  yDot : Inport  Port=2
  Constant : Constant  Value=-0.1286173633440519
  Degrees to Radians : simulink_extras/Transformations/Degrees to Radians
  Detect Change : simulink/Logic and Bit Operations/Detect Change  vinit=0  OutDataTypeStr=boolean
  Display : Display
  Gain : Gain  Gain=-1
  Gain1 : Gain
  Integrator2 : Integrator  ExternalReset=rising  LimitOutput=on  UpperSaturationLimit=10  LowerSaturationLimit=-10
  KD_dot : Gain  Gain=0
  KI_dot : Gain
  KP_dot : Gain  Gain=1.1
  Mux2 : Mux
  Radians to Degrees2 : simulink_extras/Transformations/Radians to Degrees
  Radians to Degrees7 : simulink_extras/Transformations/Radians to Degrees
  Sum2 : Sum  Inputs=|+-
  Sum3 : Sum  Inputs=3
  Sum4 : Sum  Inputs=|+-
  control terms : Scope
  filtered derivative : TransferFcn  Numerator=[100 0]  Denominator=[1 100]
  selected mission : Constant  Value=selected_mission  OutDataTypeStr=double
  theta_tether tracking : Scope  NumInputPorts=2
  y axis velocity tracking : Scope  NumInputPorts=2
  roll setpoint : Outport  VectorParamsAs1DForOutWhenUnconnected=on
  wires:
  Sum2/1 -> filtered derivative/1, KI_dot/1, KP_dot/1
  y/1 -> Radians to Degrees7/1
  Sum4/1 -> Gain1/1  "velocity setpoint (m/s)"
  yDot/1 -> Radians to Degrees2/1  "velocity"
  filtered derivative/1 -> KD_dot/1
  KD_dot/1 -> Mux2/3, Sum3/3  "D"
  KP_dot/1 -> Mux2/1, Sum3/1  "P"
  Integrator2/1 -> Mux2/2, Sum3/2  "I"
  Sum3/1 -> Mux2/4, Gain/1  "total"
  KI_dot/1 -> Integrator2/1
  Radians to Degrees7/1 -> Sum4/2, theta_tether tracking/2  "yzTether"
  Gain/1 -> Display/1, Degrees to Radians/1  "roll_setPoint"
  Mux2/1 -> control terms/1  "yz_controlInputs"
  Radians to Degrees2/1 -> y axis velocity tracking/2, Sum2/2  "yzTetherDot"
  Degrees to Radians/1 -> roll setpoint/1
  Constant/1 -> Sum4/1, theta_tether tracking/1  "yzTetherSetpoint"
  Gain1/1 -> y axis velocity tracking/1, Sum2/1
  Detect Change/1 -> Integrator2/2
  selected mission/1 -> Detect Change/1  "run_mission"

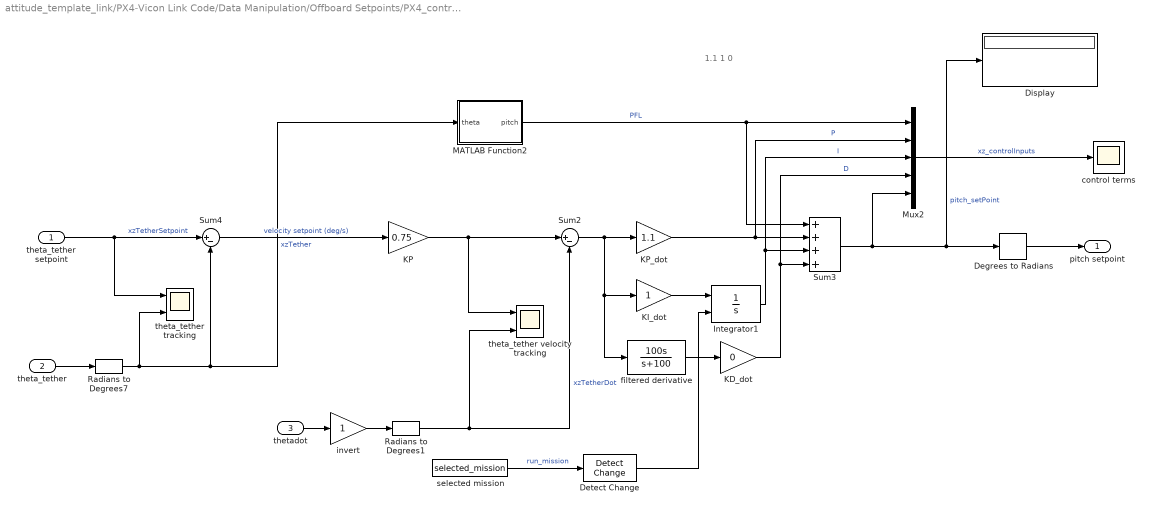
== system attitude_template_link/PX4-Vicon Link Code/Data Manipulation/Offboard Setpoints/PX4_controller/Cutter Module Position Controller/theta_tether Controller ==
  note: 1.1 1 0
  theta_tether setpoint : Inport
  theta_tether : Inport  Port=2
  thetadot : Inport  Port=3
  Degrees to Radians : simulink_extras/Transformations/Degrees to Radians
  Detect Change : simulink/Logic and Bit Operations/Detect Change  vinit=0  OutDataTypeStr=boolean
  Display : Display
  Integrator1 : Integrator  ExternalReset=rising  LimitOutput=on  UpperSaturationLimit=10  LowerSaturationLimit=-10
  KD_dot : Gain  Gain=0
  KI_dot : Gain
  KP : Gain  Gain=0.75
  KP_dot : Gain  Gain=1.1
  MATLAB Function2 : MATLAB Function  TreatAsAtomicUnit=on
  Mux2 : Mux  Inputs=5
  Radians to Degrees1 : simulink_extras/Transformations/Radians to Degrees
  Radians to Degrees7 : simulink_extras/Transformations/Radians to Degrees
  Sum2 : Sum  Inputs=|+-
  Sum3 : Sum  Inputs=4
  Sum4 : Sum  Inputs=|+-
  control terms : Scope
  filtered derivative : TransferFcn  Numerator=[100 0]  Denominator=[1 100]
  invert : Gain
  selected mission : Constant  Value=selected_mission  OutDataTypeStr=double
  theta_tether tracking : Scope  NumInputPorts=2
  theta_tether velocity tracking : Scope  NumInputPorts=2
  pitch setpoint : Outport  VectorParamsAs1DForOutWhenUnconnected=on
  wires:
  theta_tether setpoint/1 -> theta_tether tracking/1, Sum4/1  "xzTetherSetpoint"
  theta_tether/1 -> Radians to Degrees7/1
  thetadot/1 -> invert/1
  Radians to Degrees1/1 -> Sum2/2, theta_tether velocity tracking/2  "xzTetherDot"
  KI_dot/1 -> Integrator1/1
  Sum2/1 -> filtered derivative/1, KI_dot/1, KP_dot/1
  KP_dot/1 -> Mux2/2, Sum3/2  "P"
  Integrator1/1 -> Mux2/3, Sum3/3  "I"
  Sum3/1 -> Mux2/5, Degrees to Radians/1, Display/1  "pitch_setPoint"
  invert/1 -> Radians to Degrees1/1
  Radians to Degrees7/1 -> MATLAB Function2/1(theta), Sum4/2, theta_tether tracking/2  "xzTether"
  Mux2/1 -> control terms/1  "xz_controlInputs"
  filtered derivative/1 -> KD_dot/1
  MATLAB Function2/1(pitch) -> Sum3/1, Mux2/1  "PFL"
  KD_dot/1 -> Mux2/4, Sum3/4  "D"
  Degrees to Radians/1 -> pitch setpoint/1
  selected mission/1 -> Detect Change/1  "run_mission"
  Detect Change/1 -> Integrator1/2
  Sum4/1 -> KP/1  "velocity setpoint (deg/s)"
  KP/1 -> theta_tether velocity tracking/1, Sum2/1

== system attitude_template_link/PX4-Vicon Link Code/Data Manipulation/Offboard Setpoints/PX4_controller/Mission Selector/Switch Case Action Subsystem1 ==
  In1 : Inport
  Action Port : ActionPort  ActionPortLabel=case [ 2 ]:
  Out1 : Outport
  wires:
  In1/1 -> Out1/1

== system attitude_template_link/PX4-Vicon Link Code/Data Manipulation/Offboard Setpoints/PX4_controller/Mission Selector/Switch Case Action Subsystem2 ==
  In1 : Inport
  Action Port : ActionPort  ActionPortLabel=case [ 1 ]:
  Out1 : Outport
  wires:
  In1/1 -> Out1/1

== system attitude_template_link/PX4-Vicon Link Code/Data Manipulation/Offboard Setpoints/PX4_controller/Mission Selector/Switch Case Action Subsystem3 ==
  In1 : Inport
  Action Port : ActionPort  ActionPortLabel=case [ 3 ]:
  Out1 : Outport
  wires:
  In1/1 -> Out1/1

== matlab function attitude_template_link/PX4-Vicon Link Code/Data Manipulation/Manipulation_Object1/Co-ord shift ==
  data: u input; y output; orgin_TM input; tether_length input
function y = fcn(u, orgin_TM, tether_length)
%shfit origin of cooridnate system to tether attachment point on parent
%drone
orgin_TM(3) = orgin_TM(3) + tether_length;

for i = 1:3
u(i) = u(i) - orgin_TM(i);
end

%y=zeros(3,1);
y = u;

== matlab function attitude_template_link/PX4-Vicon Link Code/Data Manipulation/Offboard Setpoints/PX4_controller/Cutter Module Position Controller/Crosstrack error Controller/Gain ==
  data: error input; i_in input; i_out output
function i_out = fcn(error,i_in)

if(abs(error) < 0.01)
    i_out = 0;
   
else 
    i_out = 4*i_in;
    
  
    
end

== matlab function attitude_template_link/PX4-Vicon Link Code/Data Manipulation/Offboard Setpoints/PX4_controller/Sensor input conversion/MATLAB Function ==
  data: x input; theta_xz output; z input
function theta_xz  = theta_xzProjection(x,z)

theta_xz = atan(x/abs(z));

== matlab function attitude_template_link/PX4-Vicon Link Code/Data Manipulation/Offboard Setpoints/PX4_controller/Cutter Module Position Controller/Crosstrack error Controller/Gain1 ==
  data: error input; i_in input; i_out output
function i_out = fcn(error,i_in)

if(abs(error) < 0.01)
    i_out = 0;
   
else 
    i_out = i_in;
    
  
    
end

== matlab function attitude_template_link/PX4-Vicon Link Code/Data Manipulation/Offboard Setpoints/PX4_controller/Sensor input conversion/MATLAB Function1 ==
  data: z input; y input; theta_yz output
function theta_yz  = theta_yzProjection(z,y)

theta_yz = atan(y/abs(z));

== matlab function attitude_template_link/PX4-Vicon Link Code/Data Manipulation/Offboard Setpoints/MATLAB Function ==
  data: Pitch input; Roll input; Yaw input; Quaternion output
function Quaternion = fcn(Pitch, Roll, Yaw)

Quaternion = eul2quat([Yaw, Pitch, Roll]);

== matlab function attitude_template_link/PX4-Vicon Link Code/Data Manipulation/Offboard Setpoints/PX4_controller/Cutter Module Position Controller/theta_tether Controller/MATLAB Function2 ==
  data: theta input; pitch output
function pitch = fcn(theta)
% pitch = 7e-05*theta^4 - 0.0037*theta^3 + 0.0719*theta^2 + 0.2475*theta + 0.6532;

% TBody = 6.9;
TBody = 3.355;
m = 0.667;
g = 9.81;

if abs(theta) < 30
    pitch =  asind(m*g * sind(theta)/TBody) - theta;
else
    pitch = 50*sign(theta);
end
